simulink model "fun1"  (R2012b)
settings: Solver=ode45  StartTime=0.0  StopTime=200  RelTol=1e-3
settings Model: Creator=ZhouHaoyu  LastModifiedBy=ZhouHaoyu
settings DataIOCC: ExternalInput=[t, Alt,Vel]  LoadExternalInput=on

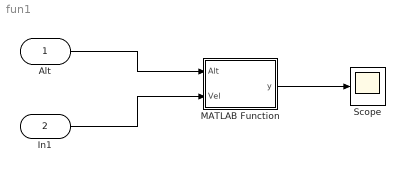
== system fun1 ==
  "Alt " : Inport
  In1 : Inport  Port=2
  MATLAB Function : MATLAB Function  TreatAsAtomicUnit=on
  Scope : Scope
  wires:
  MATLAB Function/1(y) -> Scope/1
  "Alt "/1 -> MATLAB Function/1(Alt)
  In1/1 -> MATLAB Function/2(Vel)

== matlab function fun1/MATLAB Function ==
  data: Alt input; y output; Vel input
function y = fcn(Alt,Vel)
%% 函数实现降落伞自动打开功能
%% 定义
%%Alt表示飞行器此刻所处高度
%%Vel表示飞行器此刻的速度
%%输出1表示降落伞打开，输出0表示降落伞关闭
%% 实现
y = 0;
if(Alt<=17000)&&(Vel<=503.8)
    y=1;
end
if(Alt<=6500)
    y=1;
end
end
